simulink model "example11_2"  (R2022b)
settings: Solver=FixedStepAuto  StartTime=0.0  StopTime=100  FixedStep=0.01  RelTol=1e-3
InitFcn:
  | example11_2_param;
values from neighbouring files (symbols this model uses):
  A = [0 1 0;0 0 1;0 -24 -10]    [example11_2_param.m]
  A11 = 0    [example11_2_param.m]
  A12 = [1 0]    [example11_2_param.m]
  A21 = [0; 0]    [example11_2_param.m]
  A22 = [0 1; -24 -10]    [example11_2_param.m]
  B = [0 ; 10 ; -80]    [example11_2_param.m]
  B1 = 0    [example11_2_param.m]
  B2 = [10; -80]    [example11_2_param.m]
  C = [1 0 0]    [example11_2_param.m]
  eta0 = [0; 0]    [example11_2_param.m]
  G = acker(A22',A12',[-10; -10])'    [example11_2_param.m]
  K = place(A,B,[-1+2i; -1 - 2i; -5])    [example11_2_param.m]
settings Model: LastModifiedBy=vcichella
settings DebuggingCC: UnconnectedInputMsg=warning  UnconnectedOutputMsg=warning  UnconnectedLineMsg=warning
settings ModelReferenceCC: EnableRefExpFcnMdlSchedulingChecks=on
settings RTWCC: DLArmComputeVersion=19.05

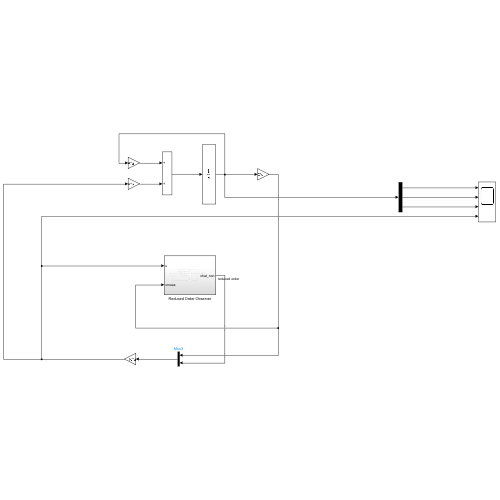
[thumbnail: Simulink's stored preview of the top-level diagram]
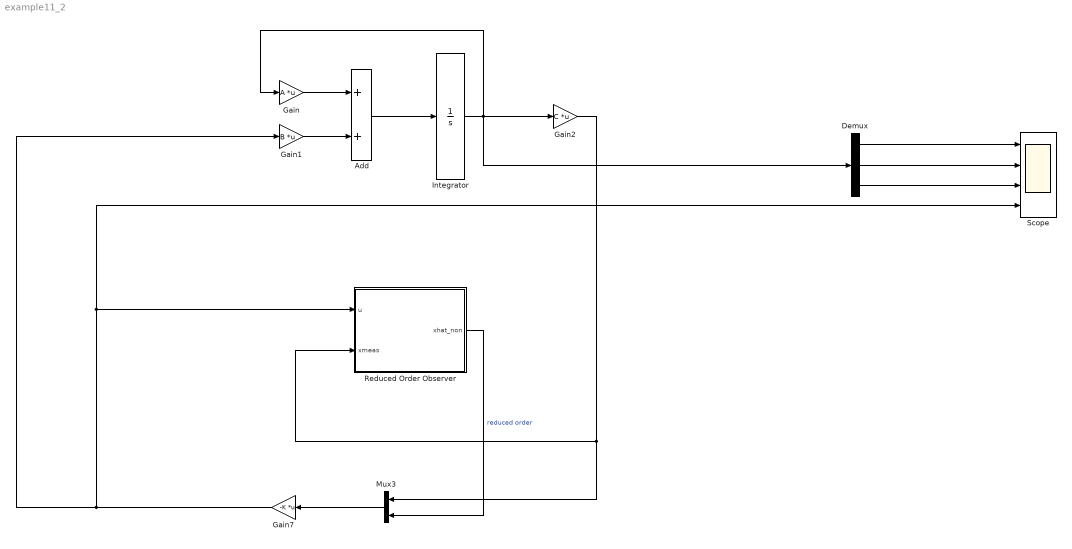
== system example11_2 ==
  Add : Sum
  Demux : Demux  Outputs=3
  Gain : Gain  Gain=A  Multiplication=Matrix(K*u)
  Gain1 : Gain  Gain=B  Multiplication=Matrix(K*u)
  Gain2 : Gain  Gain=C  Multiplication=Matrix(K*u)
  Gain7 : Gain  Gain=-K  Multiplication=Matrix(K*u)
  Integrator : Integrator  InitialCondition=[1;0;0]
  Mux3 : Mux  Inputs=2
  Reduced Order Observer : Subsystem
  Scope : Scope  NumInputPorts=4
  wires:
  Add/1 -> Integrator/1
  Gain/1 -> Add/1
  Gain1/1 -> Add/2
  Integrator/1 -> Demux/1, Gain2/1, Gain/1
  Demux/1 -> Scope/1
  Demux/2 -> Scope/2
  Demux/3 -> Scope/3
  Gain7/1 -> Gain1/1, Reduced Order Observer/1(u), Scope/4
  Gain2/1 -> Mux3/1, Reduced Order Observer/2(xmeas)
  Mux3/1 -> Gain7/1
  Reduced Order Observer/1(xhat_non) -> Mux3/2  "reduced order"

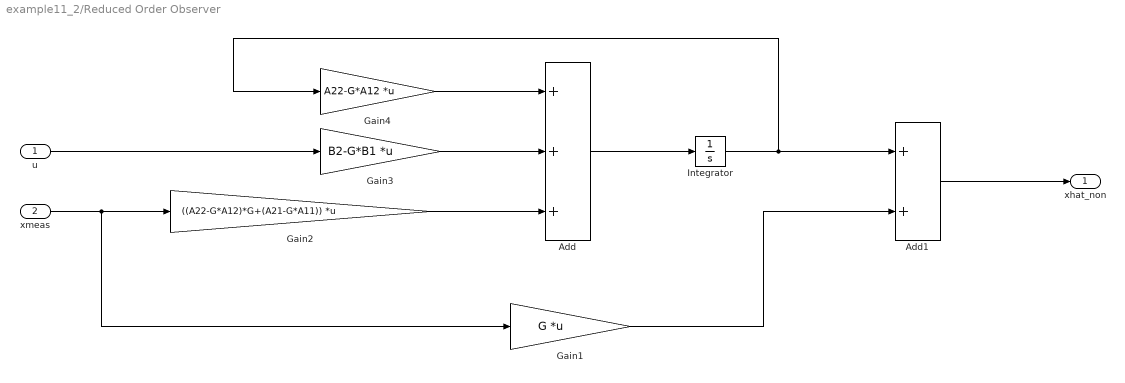
== system example11_2/Reduced Order Observer ==
  u : Inport
  xmeas : Inport  Port=2
  Add : Sum  Inputs=+++
  Add1 : Sum
  Gain1 : Gain  Gain=G  Multiplication=Matrix(K*u)
  Gain2 : Gain  Gain=((A22-G*A12)*G+(A21-G*A11))  Multiplication=Matrix(K*u)
  Gain3 : Gain  Gain=B2-G*B1  Multiplication=Matrix(K*u)
  Gain4 : Gain  Gain=A22-G*A12  Multiplication=Matrix(K*u)
  Integrator : Integrator  InitialCondition=eta0
  xhat_non : Outport
  wires:
  Gain3/1 -> Add/2
  u/1 -> Gain3/1
  Gain2/1 -> Add/3
  xmeas/1 -> Gain1/1, Gain2/1
  Gain4/1 -> Add/1
  Add/1 -> Integrator/1
  Integrator/1 -> Add1/1, Gain4/1
  Add1/1 -> xhat_non/1
  Gain1/1 -> Add1/2
